simulink model "robot2"  (R2016b)
settings: Solver=ode45  StartTime=0.0  StopTime=20  RelTol=1e-3  EnableMultiTasking=on
PreLoadFcn:
  | fprintf('*** Loading Puma560 model to workspace\n');
  | mdl_puma560
values from neighbouring files (symbols this model uses):
  q1 = q    [qianquJ.m]
  roldm = SerialLink([L1,L2,L3,L4],'name','oldm')    [myikine.m]
undefined symbols (not defined in the file or in its folder): DiscIntNeverNeededParam, transl
libraries: roblocks x6, simulink x1
settings Model: ExtModeTrigMode=oneshot  ExtModeArmWhenConnect=off  Creator=pic  LastModifiedBy=yehoo
settings DataIOCC: SaveFormat=Array  SignalLoggingSaveFormat=ModelDataLogs
settings OptimizationCC: BlockReduction=off  BooleanDataType=off  ExpressionDepthLimit=2147483647  InitFltsAndDblsToZero=on  LifeSpan=inf
settings DebuggingCC: SaveWithParameterizedLinksMsg=none  UnderspecifiedInitializationDetection=Classic  MergeDetectMultiDrivingBlocksExec=none  SignalResolutionControl=TryResolveAllWithWarning  MultiTaskDSMMsg=warning  MultiTaskCondExecSysMsg=none  FcnCallInpInsideContextMsg=warning  AllowSymbolicDim=off  StateNameClashWarn=warning  SFUnexpectedBacktrackingDiag=warning  SFNoUnconditionalDefaultTransitionDiag=warning  SFExecutionAtInitializationDiag=none
settings HardwareCC: ProdBitPerPointer=32  ProdBitPerSizeT=32  ProdBitPerPtrDiffT=32  ProdLargestAtomicFloat=None  ProdIntDivRoundTo=Undefined  ProdEndianess=Unspecified  ProdWordSize=32  ProdHWDeviceType=32-bit Generic  TargetBitPerPointer=64  TargetBitPerSizeT=64  TargetBitPerPtrDiffT=64  TargetLongLongMode=on  TargetIntDivRoundTo=Zero  TargetEndianess=LittleEndian  TargetWordSize=64  TargetHWDeviceType=MATLAB Host  ProdEqTarget=off
settings ModelReferenceCC: PropagateSignalLabelsOutOfModel=off
settings GRTTargetCC: TargetLangStandard=C89/C90 (ANSI)  ModelReferenceCompliant=off  CompOptLevelCompliant=off  GeneratePreprocessorConditionals=Disable all  CombineOutputUpdateFcns=off  MatFileLogging=off  GRTInterface=on
settings ConfigComp: CovMetricSettings=dw  CovHtmlReporting=on  CovSaveCumulativeToWorkspaceVar=on  CovSaveSingleToWorkspaceVar=on  CovExternalEMLEnable=off

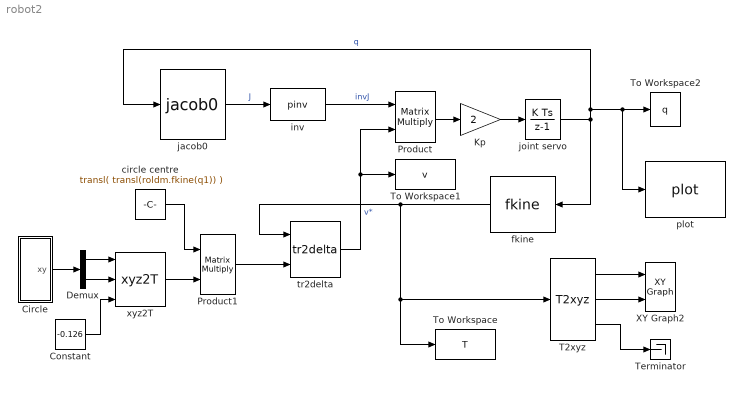
== system robot2 ==
  Circle : Subsystem  mask{radius=0.1, freq=0.1}
      mask prompts: freq "Frequency (rev/s)"
  Constant : Constant  Value=-0.126
  Demux : Demux  Outputs=2
  Kp : Gain  Gain=2  SaturateOnIntegerOverflow=on  OutDataTypeStr=Inherit: Same as input  ParamDataTypeStr=Inherit: Same as input
  Product : Product  Multiplication=Matrix(*)  SaturateOnIntegerOverflow=on  RndMeth=Zero  InputSameDT=on  OutDataTypeStr=Inherit: Same as first input
  Product1 : Product  Multiplication=Matrix(*)  SaturateOnIntegerOverflow=on  RndMeth=Zero  InputSameDT=on  OutDataTypeStr=Inherit: Same as first input
  T2xyz : roblocks/Toolbox/T2xyz
  Terminator : Terminator
  To Workspace : ToWorkspace  VariableName=T  SampleTime=-1
  To Workspace1 : ToWorkspace  VariableName=v  SampleTime=-1
  To Workspace2 : ToWorkspace  VariableName=q  SampleTime=-1
  XY Graph2 : simulink/Sinks/XY Graph  xmin=-0.5  xmax=0.5  ymin=0.5  ymax=1  st=-1
  circle centre : Constant  Value=transl( transl(roldm.fkine(q1)) )
  fkine : roblocks/Arm/fkine  robot=roldm
  inv : MATLABFcn  MATLABFcn=pinv  Output1D=off
  "jacob0 " : roblocks/Arm/jacob0   robot=roldm
      link override MATLAB Fcn: MATLABFcn=jacob0(robot,u)
  joint servo : DiscreteIntegrator  InitialCondition=q1'  InitialConditionSetting=State (most efficient)  SampleTime=0.05  ICPrevOutput=DiscIntNeverNeededParam  ICPrevScaledInput=DiscIntNeverNeededParam
  plot : roblocks/Arm/plot  robot=roldm  fps=25  holdplot=on
  tr2delta : roblocks/Toolbox/tr2delta
  xyz2T : roblocks/Toolbox/xyz2T
  wires:
  joint servo/1 -> plot/1, To Workspace2/1, "jacob0 "/1, fkine/1  "q"
  T2xyz/1 -> XY Graph2/1
  T2xyz/2 -> XY Graph2/2
  tr2delta/1 -> Product/2, To Workspace1/1  "v*"
  Demux/1 -> xyz2T/1
  "jacob0 "/1 -> inv/1  "J"
  Product/1 -> Kp/1
  inv/1 -> Product/1  "invJ"
  Kp/1 -> joint servo/1
  Demux/2 -> xyz2T/2
  Circle/1(xy) -> Demux/1
  Constant/1 -> xyz2T/3
  fkine/1 -> tr2delta/1, To Workspace/1, T2xyz/1
  xyz2T/1 -> Product1/2
  T2xyz/3 -> Terminator/1
  Product1/1 -> tr2delta/2
  circle centre/1 -> Product1/1

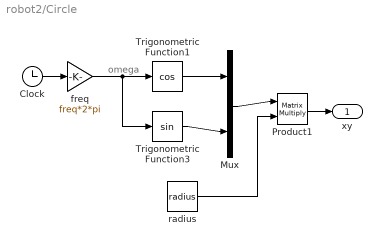
== system robot2/Circle ==
  note: omega
  Clock : Clock
  Mux : Mux  Inputs=2
  Product1 : Product  Multiplication=Matrix(*)  RndMeth=Zero
  Trigonometric Function1 : Trigonometry  Operator=cos
  Trigonometric Function3 : Trigonometry
  freq : Gain  Gain=freq*2*pi
  radius : Constant  Value=radius
  xy : Outport
  wires:
  freq/1 -> Trigonometric Function3/1, Trigonometric Function1/1
  Product1/1 -> xy/1
  Clock/1 -> freq/1
  radius/1 -> Product1/2
  Mux/1 -> Product1/1
  Trigonometric Function1/1 -> Mux/1
  Trigonometric Function3/1 -> Mux/2
